simulink library "Lib_Turbo_StaticCalc_TMATS_org"  (Simulink 10.0)
settings: Solver=ode45  StartTime=0.0  StopTime=10.0  RelTol=1e-3  EnableMultiTasking=on
Description:
  | Thomas Modules
settings Model: Creator=jwchapm2  LastModifiedBy=annonymous

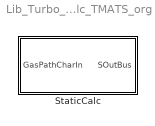
== system Lib_Turbo_StaticCalc_TMATS_org ==
  StaticCalc : Subsystem  mask(T-MATS: Static Calculation Library Block){ST_M=off, Ath_M=100, MN_M=0.5, X_FARVec_M=[0; 0.0050; 0.0100; 0.0150; 0.0200; 0.0250; 0.0300], Y_TtVec_M=[300 10000], T_RtArray_M=[0.0686;    0.0686;    0.0686;    0.0686;    0.0686;    0.0686;    0.0686], T_gammaArray_M=[ 1.4 1.4 1.4 1.4 1.4 1.4 1.4; 1.4 1.4 1.4 1.4 1.4 1.4 1.4]}
      mask prompts: ST_M "ST_M - Solve Type ( unchecked - Assumed Ath, checked - Assumed MN)"; Ath_M "Ath_M - Assumed throat Area, Ath [in^2]"; MN_M "MN_M - Assumed Mach Number (will use as initial guess with asusmed Ath)"; X_FARVec_M "X_FARVec_M - Fuel to Air Ratio Vector (X-axis) (cx1)"; Y_TtVec_M "Y_TtVec_M - Total Temperature Vector (Y-axis for Gamma calc)(dx1)"; T_RtArray_M "T_RtArray_M - Gas Constant, R, Array (R = f(FAR))(cx1)"; T_gammaArray_M "T_gammaArray_M - Gamma Array (Gamma = f(Tt,FAR))(dxc)"
      mask help: This Block calculates static pressure and temperature from an input flow stream and either an assumed throat area or mach number.
      mask Help: web(which('Turbo_TMATS_StCalc.html'),'-helpbrowser')
      mask Callback ST_M: MSK_SEC_Enables_TMATS('ST_M',[2],'dis')

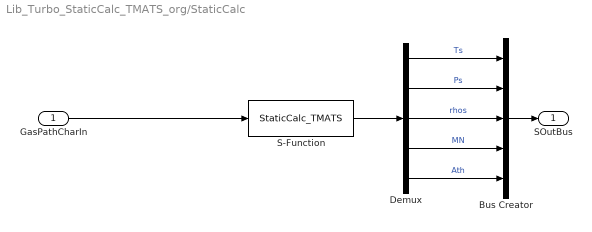
== system Lib_Turbo_StaticCalc_TMATS_org/StaticCalc ==
  GasPathCharIn : Inport
  Bus Creator : BusCreator  Inputs=5
  Demux : Demux  Outputs=5
  S-Function : S-Function  FunctionName=StaticCalc_TMATS  Parameters=Ath_M, MN_M, ST_M, X_FARVec_M, T_RtArray_M, Y_TtVec_M, T_gammaArray_M, gcb  SFunctionModules='t2hc_TMATS sp2tc_TMATS pt2sc_TMATS interp1Ac_TMATS interp2Ac_TMATS PcalcStat_TMATS functions_TMATS'  SFunctionDeploymentMode=off  EnableBusSupport=off
  SOutBus : Outport
  wires:
  GasPathCharIn/1 -> S-Function/1
  S-Function/1 -> Demux/1
  Demux/1 -> Bus Creator/1  "Ts"
  Demux/2 -> Bus Creator/2  "Ps"
  Demux/3 -> Bus Creator/3  "rhos"
  Demux/5 -> Bus Creator/5  "Ath"
  Demux/4 -> Bus Creator/4  "MN"
  Bus Creator/1 -> SOutBus/1
